simulink library "Flow_Diverter"  (Simulink 8.2)
settings: Solver=ode45  StartTime=0.0  StopTime=10.0  RelTol=1e-3
undefined symbols (not defined in the file): DPConstant, DPLinear, DPQuadratic, ID, MassFlow
settings Model: Creator=lena.frank  LastModifiedBy=drhf

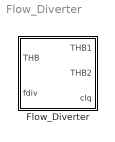
== system Flow_Diverter ==
  Flow_Diverter : Subsystem  mask(flow diverter, fixed rate){}
      mask help:
      | The block diverts an incoming massflow according to:
      | mdot1 = mdot * fdiv
      | mdot2 = mdot * (1-fdiv)
      | fdiv is limited to the range [0..1]
      mask Help: web(fullfile(path_carnot('help'),'Flow_Diverter.html'),'-helpbrowser')
      mask Display: plot(0,-5,120,65,[20 45 20 20],[20 30 40 20],[45 70 70 45],[30 20 40 30],[45 35 55 45],[30 10 10 30])

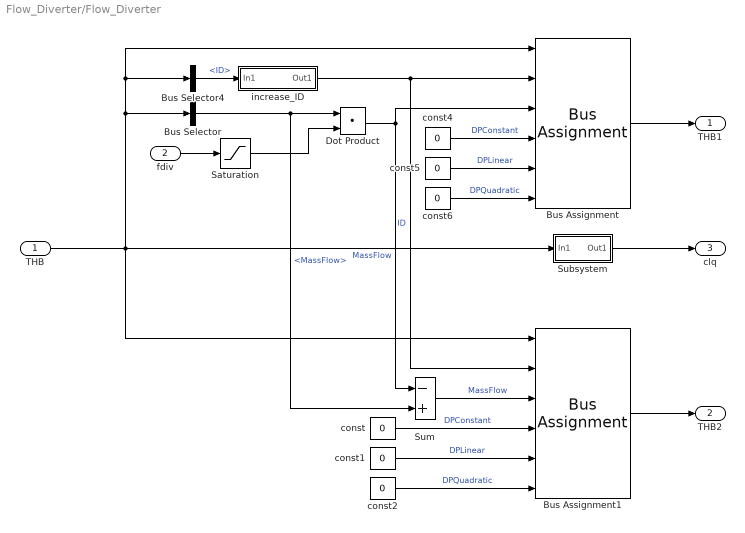
== system Flow_Diverter/Flow_Diverter ==
  THB : Inport
  fdiv : Inport  Port=2
  Bus Assignment : BusAssignment  AssignedSignals=ID,MassFlow,DPConstant,DPLinear,DPQuadratic
  Bus Assignment1 : BusAssignment  AssignedSignals=ID,MassFlow,DPConstant,DPLinear,DPQuadratic
  Bus Selector : BusSelector  OutputSignals=MassFlow
  Bus Selector4 : BusSelector  OutputSignals=ID
  Dot Product : DotProduct  InputSameDT=on  OutDataTypeStr=Inherit: Inherit via internal rule
  Saturation : Saturate  UpperLimit=1  LowerLimit=0
  Subsystem : Subsystem
  Sum : Sum  Inputs=-+  SaturateOnIntegerOverflow=on  InputSameDT=on  OutDataTypeStr=Inherit: Same as first input
  const{,1..2,4..6} (6 alike) : Constant  Value=0
  increase_ID : Subsystem
  THB1 : Outport
  THB2 : Outport  Port=2
  clq : Outport  Port=3
  wires:
  const2/1 -> Bus Assignment1/6  "DPQuadratic"
  const1/1 -> Bus Assignment1/5  "DPLinear"
  Saturation/1 -> Dot Product/2
  Sum/1 -> Bus Assignment1/3  "MassFlow"
  Bus Selector/1 -> Dot Product/1, Sum/2  "<MassFlow>"
  const/1 -> Bus Assignment1/4  "DPConstant"
  THB/1 -> Bus Selector/1, Bus Assignment/1, Bus Selector4/1, Bus Assignment1/1, Subsystem/1(In1)
  fdiv/1 -> Saturation/1
  Dot Product/1 -> Sum/1, Bus Assignment/3  "MassFlow"
  Bus Selector4/1 -> increase_ID/1(In1)  "<ID>"
  increase_ID/1(Out1) -> Bus Assignment/2, Bus Assignment1/2  "ID"
  const6/1 -> Bus Assignment/6  "DPQuadratic"
  const5/1 -> Bus Assignment/5  "DPLinear"
  const4/1 -> Bus Assignment/4  "DPConstant"
  Bus Assignment/1 -> THB1/1
  Bus Assignment1/1 -> THB2/1
  Subsystem/1(Out1) -> clq/1

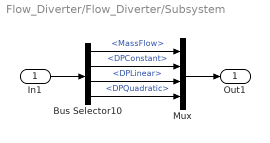
== system Flow_Diverter/Flow_Diverter/Subsystem ==
  In1 : Inport
  Bus Selector10 : BusSelector  OutputSignals=MassFlow,DPConstant,DPLinear,DPQuadratic
  Mux : Mux
  Out1 : Outport
  wires:
  Bus Selector10/1 -> Mux/1  "<MassFlow>"
  Bus Selector10/2 -> Mux/2  "<DPConstant>"
  Bus Selector10/3 -> Mux/3  "<DPLinear>"
  Bus Selector10/4 -> Mux/4  "<DPQuadratic>"
  In1/1 -> Bus Selector10/1
  Mux/1 -> Out1/1

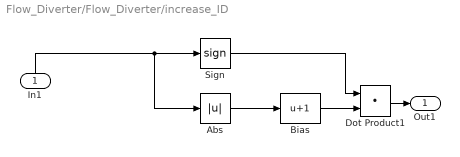
== system Flow_Diverter/Flow_Diverter/increase_ID ==
  In1 : Inport
  Abs : Abs
  Bias : Bias  Bias=1
  Dot Product1 : DotProduct  InputSameDT=on  OutDataTypeStr=Inherit: Inherit via internal rule
  Sign : Signum
  Out1 : Outport
  wires:
  Bias/1 -> Dot Product1/2
  Sign/1 -> Dot Product1/1
  Abs/1 -> Bias/1
  Dot Product1/1 -> Out1/1
  In1/1 -> Sign/1, Abs/1
